simulink library "ddm"  (R2021b)
settings: Solver=VariableStepAuto  StartTime=0.0  StopTime=10.0  RelTol=1e-3
undefined symbols (not defined in the file or in its folder): ADDM_FrTMTqDev_X_Nm, ADDM_RrTMTqDev_X_Nm, ENUM_ADASACCSTA_ERROR, ENUM_ADASACCSTA_OFF, ENUM_ADASACCSTA_STANDBY, ENUM_ALLOWMOV_ALLOWREADY, ENUM_APS, ENUM_BRKSTA_ERROR, ENUM_BRKSTA_OFF, ENUM_BRKSTA_ON, ENUM_BRKSW_INVALID, ENUM_BRKSW_OFF, ENUM_BRKSW_ON, ENUM_CHGPREACTERRSTA_OBCPRE, ENUM_DCDCFAULTSTA_ANYFAULTLV1, ENUM_DCDCFAULTSTA_ANYFAULTLV2, ENUM_DRIVETRAIN_AWD, ENUM_DRIVETRAIN_FWD, ENUM_DRIVETRAIN_RWD, ENUM_EDUDRTSTA_NORMAL, ENUM_EPBSTA_APPLIED, ENUM_EPBSTA_RELEASED, ENUM_ESCAPSSta_APSUNAVAILABLE, ENUM_GEARACTUALPOSN_INVALID, ENUM_GEARACTUALPOSN_P, ENUM_HVBATTREADYPRE_READY, ENUM_MCUWARN_LV0, ENUM_MCUWARN_LV1, ENUM_MCUWARN_LV2, ENUM_MCUWARN_LV3, ENUM_MCUWARN_NOERROR, ENUM_OBCFAULTSTA_ANYFAULT, ENUM_PAS_R2F2, ENUM_PDFAULT_BATTPDFAIL, ENUM_PDFAULT_DCDCDISABLE, ENUM_PDFAULT_MCUDISABLE, ENUM_PDFAULT_MCUDISCHRG, ENUM_POWERSTA_OFF, ENUM_POWERSTA_ON, ENUM_POWERSTA_READY, ENUM_POWERSTA_STANDBY, ENUM_PRESSINDI_LOW, ENUM_PUFAULT_BATTUPFAIL, ENUM_PUFAULT_DCDCENABLEFAIL, ENUM_PUFAULT_PRECHRGCHKFAIL, ENUM_PUFAULT_SAFETYCHKFAIL, ENUM_PUSTATE_COMPLETED, ENUM_PWRSTASW_OFF, ENUM_PWRSTASW_OFFA, ENUM_PWRSTASW_OFFCHVCHRG, ENUM_PWRSTASW_OFFCLVCHRG, ENUM_PWRSTASW_ON, ENUM_PWRSTASW_ONHVCHRG, ENUM_PWRSTASW_READY, ENUM_PWRSTASW_STANDBY, ENUM_RAPSErrWarnSta_NORMAL, ENUM_RAPSErrWarnSta_RAPSERRLV1, ENUM_SHIFTCOMMAND_P, ENUM_SHIFTERERRSTA_PBUTTONFAILURE, ENUM_VEHMALFUNLV_2ND ... (+463)
libraries: hcu_lib x529, $bdroot x5, simulink x4
(part 6 of 25)

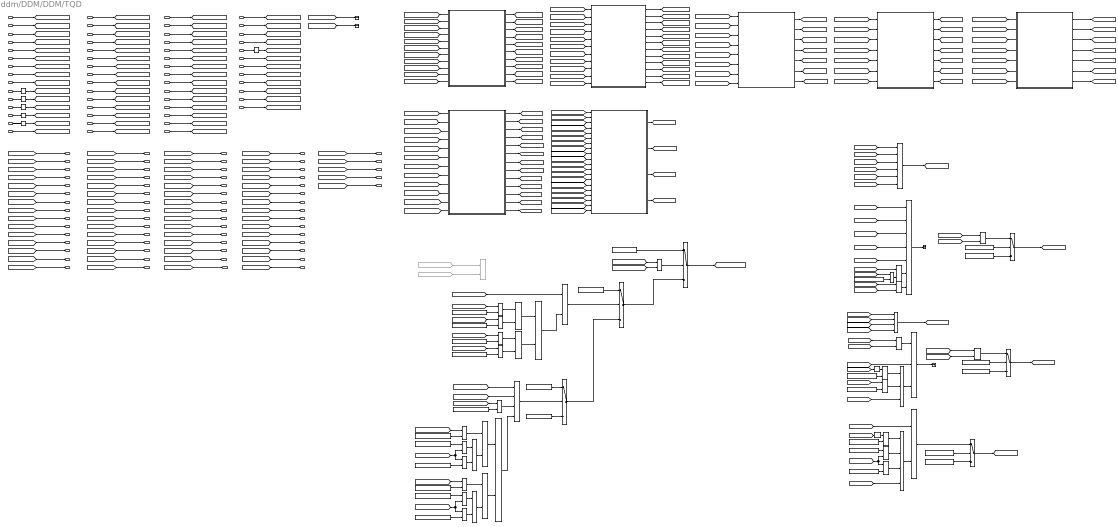
== system ddm/DDM/DDM/TQD ==
  note: VDDM_EPB1Err_flg
  note: Shifeter Error lamp Signal
  note: Three-electrical warning
  note: Warning lamp Signal
  note: RAPS Signal error
  VPMM_SysPwrSta_enum : Inport
  VINP_AccelPedal1Vol_V : Inport  Port=2
  VINP_AccelPedal2Vol_V : Inport  Port=3
  VDHP_EAPS12RangeSta_enum : Inport  Port=4
  VDHP_EAPCRBAD_flg : Inport  Port=5
  task_time_s : Inport  Port=6
  DTC_clear_request : Inport  Port=7
  No_CAN3_BUS_OFF : Inport  Port=8
  No_CAN1_BUS_OFF : Inport  Port=9
  VINP_CANMsgValidMCUNF1_flg : Inport  Port=10
  VINP_CANMsgValidMCUNR1_flg : Inport  Port=11
  VINP_CANMsgValidShifter1_flg : Inport  Port=12
  VINP_CANMsgValidESC1_flg : Inport  Port=13
  VINP_CANMsgValidESC5_flg : Inport  Port=14
  VDDM_MCUNF1RCErr_flg : Inport  Port=15
  VDDM_MCUNF1CSErr_flg : Inport  Port=16
  VDDM_MCUNR1RCErr_flg : Inport  Port=17
  VDDM_MCUNR1CSErr_flg : Inport  Port=18
  VDDM_Shifter1RCErr_flg : Inport  Port=19
  VDDM_Shifter1CSErr_flg : Inport  Port=20
  VDDM_ESC1RCErr_flg : Inport  Port=21
  VDDM_ESC1CSErr_flg : Inport  Port=22
  VDDM_ESC5RCErr_flg : Inport  Port=23
  VDDM_ESC5CSErr_flg : Inport  Port=24
  VINP_FrEDUDrtStaNidec_flg : Inport  Port=25
  VINP_VehSpeed_kph : Inport  Port=26
  VINP_FrEDURealTMTqNidec_Nm : Inport  Port=27
  VTQR_FrTMTqReq_Nm : Inport  Port=28
  VINP_RrEDUDrtStaNidec_flg : Inport  Port=29
  VINP_RrEDURealTMTqNidec_Nm : Inport  Port=30
  VTQR_RrTMTqReq_Nm : Inport  Port=31
  VINP_MCUWarnFNidec_enum : Inport  Port=32
  VINP_MCUWarnRNidec_enum : Inport  Port=33
  VINP_Pedal1Ref5V_V : Inport  Port=34
  VINP_Pedal2Ref5V_V : Inport  Port=35
  VINP_HVBattSOC_pct : Inport  Port=36
  VDDM_AuxBattVolV_V : Inport  Port=37
  VTQD_ActParkRequest_flg : Inport  Port=38
  VINP_EPBSta_enum : Inport  Port=39
  VINP_ShifterHandleCmd_enum : Inport  Port=40
  VINP_BMSWarn4_flg : Inport  Port=41
  VINP_BMSWarn5_flg : Inport  Port=42
  VINP_BMSWarn6_flg : Inport  Port=43
  VINP_BMSWarn7_flg : Inport  Port=44
  VINP_BMSWarn8_flg : Inport  Port=45
  VINP_DCDCFaultSta_enum : Inport  Port=46
  VPMM_DrivetrainSelect_enum : Inport  Port=47
  VTQD_GearActualPosn_enum : Inport  Port=48
  VINP_EPBErrSta_enum : Inport  Port=49
  VINP_CANMsgValidEPB1_flg : Inport  Port=50
  VDDM_EPB1RCErr_flg : Inport  Port=51
  VDDM_EPB1CSErr_flg : Inport  Port=52
  VDHP_EAPS1BAD_flg : Inport  Port=53
  VDHP_EAPS2BAD_flg : Inport  Port=54
  VDDM_C3BMS1LCCFS_flg : Inport  Port=55
  VDDM_VCURAPSErrLv2_flg : Inport  Port=56
  VVMC_APSActive_flg : Inport  Port=57
  APS_DDM : Subsystem
  Constant : Constant  Value=KDDM_SysErrShifterErrSW_flg
  Constant1 : Constant  Value=ENUM_DRIVETRAIN_FWD
  Constant10 : Constant  Value=ENUM_MCUWARN_LV3
  Constant11 : Constant  Value=ENUM_VEHMALFUNLV_3RD
  Constant12 : Constant  Value=ENUM_VEHMALFUNLV_4TH
  Constant{13..14,18..19,88} (5 alike) : Constant  Value=ENUM_GEARACTUALPOSN_P
  Constant15 : Constant  Value=ENUM_VEHMALFUNLV_2ND
  Constant16 : Constant  Value=ENUM_VEHMALFUNLV_NORMAL
  Constant17 : Constant  Value=ENUM_DCDCFAULTSTA_ANYFAULTLV2
  Constant2 : Constant  Value=ENUM_MCUWARN_LV1
  Constant20 : Constant  Value=ENUM_GEARACTUALPOSN_INVALID
  Constant21 : Constant  Value=FALSE
  Constant22 : Constant  Value=KDDM_EPBErrPopupSW_flg
  Constant23 : Constant  Value=FALSE
  Constant24 : Constant  Value=KDDM_DisengagePFailSW_flg
  Constant25 : Constant  Value=FALSE
  Constant3 : Constant  Value=ENUM_MCUWARN_LV2
  Constant4 : Constant  Value=ENUM_DRIVETRAIN_RWD
  Constant5 : Constant  Value=ENUM_MCUWARN_LV1
  Constant6 : Constant  Value=ENUM_MCUWARN_LV2
  Constant7 : Constant  Value=ENUM_DRIVETRAIN_FWD
  Constant8 : Constant  Value=ENUM_DRIVETRAIN_RWD
  Constant9 : Constant  Value=ENUM_MCUWARN_LV3
  Delay1 : Delay  DelayLength=1
  Delay2 : Delay  DelayLength=1
  EPB : Subsystem
  ESC1_DDM : Subsystem
  ESC5_DDM : Subsystem
  Equal{,1,5,8,11,15..16} (7 alike) : RelationalOperator  Operator=~=  OutDataTypeStr=boolean  RndMeth=Simplest
  Equal{2..4,6..7,9..10,12..14} (10 alike) : RelationalOperator  Operator===  OutDataTypeStr=boolean  RndMeth=Simplest
  From112 : From  Commented=on  GotoTag=VDDM_MCUNR1NoComCFS_flg
  From176 : From  Commented=on  GotoTag=VDDM_C3BMS1LCCFS_flg
  Logical Operator{,1,3..5,8} (6 alike) : Logic  Operator=NOT  AllPortsSameDT=off  OutDataTypeStr=boolean
  Logical Operator{2,10..13} (5 alike) : Logic  AllPortsSameDT=off  OutDataTypeStr=boolean
  Logical Operator6 : Logic  Inputs=3  AllPortsSameDT=off  OutDataTypeStr=boolean
  Logical Operator7 : Logic  Operator=OR  Inputs=4  AllPortsSameDT=off  OutDataTypeStr=boolean
  Logical Operator9 : Logic  Inputs=4  AllPortsSameDT=off  OutDataTypeStr=boolean
  MCU1_Nidec_DDM : Subsystem
  MCU_Nidec_DDM : Subsystem
  OR : Logic  Operator=OR  Inputs=6  AllPortsSameDT=off  OutDataTypeStr=boolean
  OR1 : Logic  Operator=OR  Inputs=7  AllPortsSameDT=off  OutDataTypeStr=boolean
  OR{4,6..7,9..10,12,14} (7 alike) : Logic  Operator=OR  AllPortsSameDT=off  OutDataTypeStr=boolean
  OR{5,8,11,13} (4 alike) : Logic  AllPortsSameDT=off  OutDataTypeStr=boolean
  OR15 : Logic  Commented=on  Operator=OR  AllPortsSameDT=off  OutDataTypeStr=boolean
  OR2 : Logic  Operator=OR  Inputs=3  AllPortsSameDT=off  OutDataTypeStr=boolean
  OR3 : Logic  Operator=OR  Inputs=4  AllPortsSameDT=off  OutDataTypeStr=boolean
  Shifter1_DDM : Subsystem
  Switch : Switch  Criteria=u2 > Threshold
  Switch1 : Switch  Criteria=u2 ~= 0
  Switch2 : Switch  Criteria=u2 ~= 0
  Switch3 : Switch  Criteria=u2 > Threshold
  Switch4 : Switch  Criteria=u2 > Threshold
  Switch6 : Switch  Criteria=u2 ~= 0
  Terminator{,1..3} (4 alike) : Terminator
  VDDM_APS1SigOoRDTC_raw32 : Outport
  VDDM_APS2SigOoRDTC_raw32 : Outport  Port=2
  VDDM_APSCorrErrDTC_raw32 : Outport  Port=3
  VDDM_MCUF1NoComDTC_raw32 : Outport  Port=4
  VDDM_MCUR1NoComDTC_raw32 : Outport  Port=5
  VDDM_Shifter1NoComDTC_raw32 : Outport  Port=6
  VDDM_ESC1NoComDTC_raw32 : Outport  Port=7
  VDDM_ESC5NoComDTC_raw32 : Outport  Port=8
  VDDM_MCUF1RCErrDTC_raw32 : Outport  Port=9
  VDDM_MCUR1RCErrDTC_raw32 : Outport  Port=10
  VDDM_MCUF1CSErrDTC_raw32 : Outport  Port=11
  VDDM_MCUR1CSErrDTC_raw32 : Outport  Port=12
  VDDM_Shifter1RCErrDTC_raw32 : Outport  Port=13
  VDDM_Shifter1CSErrDTC_raw32 : Outport  Port=14
  VDDM_ESC1RCErrDTC_raw32 : Outport  Port=15
  VDDM_ESC1CSErrDTC_raw32 : Outport  Port=16
  VDDM_ESC5RCErrDTC_raw32 : Outport  Port=17
  VDDM_ESC5CSErrDTC_raw32 : Outport  Port=18
  VDDM_FrMCUTqErrDTC_raw32 : Outport  Port=19
  VDDM_RrMCUTqErrDTC_raw32 : Outport  Port=20
  VDDM_MCUNF1NoComCFS_flg : Outport  Port=21
  VDDM_MCUNF1RCErrCFS_flg : Outport  Port=22
  VDDM_MCUNF1CSErrCFS_flg : Outport  Port=23
  VDDM_MCUNR1NoComCFS_flg : Outport  Port=24
  VDDM_MCUNR1RCErrCFS_flg : Outport  Port=25
  VDDM_MCUNR1CSErrCFS_flg : Outport  Port=26
  VDDM_ESC1NoComCFS_flg : Outport  Port=27
  VDDM_ESC1RCErrCFS_flg : Outport  Port=28
  VDDM_ESC1CSErrCFS_flg : Outport  Port=29
  VDDM_ESC5NoComCFS_flg : Outport  Port=30
  VDDM_ESC5RCErrCFS_flg : Outport  Port=31
  VDDM_ESC5CSErrCFS_flg : Outport  Port=32
  VDDM_5vAPS1OoRDTC_raw32 : Outport  Port=33
  VDDM_5vAPS2OoRDTC_raw32 : Outport  Port=34
  VDDM_EDriveSysErrTQD_flg : Outport  Port=35
  VDDM_EDriveSysErrShifterErr_flg : Outport  Port=36
  VDDM_EngagePFail_flg : Outport  Port=37
  VDDM_VehMalfunLevelTmp_enum : Outport  Port=38
  VDDM_EPBLockTODTC_raw32 : Outport  Port=39
  VDDM_EPBUnlockTODTC_raw32 : Outport  Port=40
  VDDM_EPB1NoComDTC_raw32 : Outport  Port=41
  VDDM_EPB1RCErrDTC_raw32 : Outport  Port=42
  VDDM_EPB1CSErrDTC_raw32 : Outport  Port=43
  VDDM_EPBSigErrDTC_raw32 : Outport  Port=44
  VDDM_5vAPS1OoRCFS_flg : Outport  Port=45
  VDDM_5vAPS2OoRCFS_flg : Outport  Port=46
  VDDM_APS1SigOoRCFS_flg : Outport  Port=47
  VDDM_APS2SigOoRCFS_flg : Outport  Port=48
  VDDM_APSCorrErrCFS_flg : Outport  Port=49
  VDDM_Shifter1NoComCFS_flg : Outport  Port=50
  VDDM_Shifter1RCErrCFS_flg : Outport  Port=51
  VDDM_Shifter1CSErrCFS_flg : Outport  Port=52
  VDDM_EPBSigErrCFS_flg : Outport  Port=53
  VDDM_EPB1NoComCFS_flg : Outport  Port=54
  VDDM_EPB1RCErrCFS_flg : Outport  Port=55
  VDDM_EPB1CSErrCFS_flg : Outport  Port=56
  VDDM_EPBLockTOCFS_flg : Outport  Port=57
  VDDM_EPBUnlockTOCFS_flg : Outport  Port=58
  VDDM_FrMCUNTqErrCFS_flg : Outport  Port=59
  VDDM_RrMCUNTqErrCFS_flg : Outport  Port=60
  VDDM_DisengagePFail_flg : Outport  Port=61
  VDDM_Shifter1Err_flg : Outport  Port=62
  VDDM_EPB1Err_flg : Outport  Port=63
  VDDM_ESC5Err_flg : Outport  Port=64
  VDDM_ESC1Err_flg : Outport  Port=65
  wires:
  VINP_ShifterHandleCmd_enum/1 -> [VINP_ShifterHandleCmd_enum]
  VINP_EPBSta_enum/1 -> [VINP_EPBSta_enum]
  VTQD_ActParkRequest_flg/1 -> [VTQD_ActParkRequest_flg]
  VDDM_AuxBattVolV_V/1 -> [VDDM_AuxBattVolV_V]
  VINP_HVBattSOC_pct/1 -> [VINP_HVBattSOC_pct]
  [VINP_Pedal2Ref5V_V] -> APS_DDM/7(VINP_Pedal2Ref5V_V)
  [VINP_Pedal1Ref5V_V] -> APS_DDM/6(VINP_Pedal1Ref5V_V)
  VINP_Pedal2Ref5V_V/1 -> [VINP_Pedal2Ref5V_V]
  VINP_Pedal1Ref5V_V/1 -> [VINP_Pedal1Ref5V_V]
  [VDDM_MCUNR1RCErrCFS_flg] -> MCU_Nidec_DDM/12(VDDM_MCUNR1RCErrCFS_flg)
  [VDDM_MCUNF1RCErrCFS_flg] -> MCU_Nidec_DDM/5(VDDM_MCUNF1RCErrCFS_flg)
  [VDDM_MCUNF1CSErrCFS_flg] -> MCU_Nidec_DDM/6(VDDM_MCUNF1CSErrCFS_flg)
  [No_CAN3_BUS_OFF] -> MCU_Nidec_DDM/3(No_CAN3_BUS_OFF)
  [VINP_MCUWarnFNidec_enum] -> MCU_Nidec_DDM/17(VINP_MCUWarnFNidec_enum)
  [VINP_RrEDUDrtStaNidec_flg] -> MCU_Nidec_DDM/14(VINP_RrEDUDrtStaNidec_flg)
  [VDDM_MCUNR1CSErrCFS_flg] -> MCU_Nidec_DDM/13(VDDM_MCUNR1CSErrCFS_flg)
  [VPMM_SysPwrSta_enum] -> MCU_Nidec_DDM/2(VPMM_SysPwrSta_enum)
  [VDDM_MCUNF1NoComCFS_flg] -> MCU_Nidec_DDM/4(VDDM_MCUNF1NoComCFS_flg)
  [VTQR_FrTMTqReq_Nm] -> MCU_Nidec_DDM/10(VTQR_FrTMTqReq_Nm)
  [task_time_s] -> MCU_Nidec_DDM/1(task_time_s)
  [VTQR_RrTMTqReq_Nm] -> MCU_Nidec_DDM/16(VTQR_RrTMTqReq_Nm)
  [VINP_FrEDUDrtStaNidec_flg] -> MCU_Nidec_DDM/8(VINP_FrEDUDrtStaNidec_flg)
  [VINP_FrEDURealTMTqNidec_Nm] -> MCU_Nidec_DDM/9(VINP_FrEDURealTMTqNidec_Nm)
  [VINP_RrEDURealTMTqNidec_Nm] -> MCU_Nidec_DDM/15(VINP_RrEDURealTMTqNidec_Nm)
  [DTC_clear_request] -> MCU_Nidec_DDM/19(DTC_clear_request)
  [VDDM_MCUNR1NoComCFS_flg] -> MCU_Nidec_DDM/11(VDDM_MCUNR1NoComCFS_flg)
  [VINP_MCUWarnRNidec_enum] -> MCU_Nidec_DDM/18(VINP_MCUWarnRNidec_enum)
  [VINP_VehSpeed_kph] -> MCU_Nidec_DDM/7(VINP_VehSpeed_kph)
  [VDDM_MCUNF1RCErrCFS_flg] -> VDDM_MCUNF1RCErrCFS_flg/1
  [VDDM_MCUNR1RCErrCFS_flg] -> VDDM_MCUNR1RCErrCFS_flg/1
  [VDDM_MCUNR1NoComCFS_flg] -> VDDM_MCUNR1NoComCFS_flg/1
  [VDDM_MCUNF1CSErrCFS_flg] -> VDDM_MCUNF1CSErrCFS_flg/1
  [VDDM_MCUNR1CSErrCFS_flg] -> VDDM_MCUNR1CSErrCFS_flg/1
  [VDDM_MCUNF1NoComCFS_flg] -> VDDM_MCUNF1NoComCFS_flg/1
  MCU1_Nidec_DDM/11(VDDM_MCUNR1RCErrCFS_flg) -> [VDDM_MCUNR1RCErrCFS_flg]
  MCU1_Nidec_DDM/7(VDDM_MCUNF1NoComCFS_flg) -> [VDDM_MCUNF1NoComCFS_flg]
  MCU1_Nidec_DDM/10(VDDM_MCUNR1NoComCFS_flg) -> [VDDM_MCUNR1NoComCFS_flg]
  MCU1_Nidec_DDM/9(VDDM_MCUNF1CSErrCFS_flg) -> [VDDM_MCUNF1CSErrCFS_flg]
  MCU1_Nidec_DDM/8(VDDM_MCUNF1RCErrCFS_flg) -> [VDDM_MCUNF1RCErrCFS_flg]
  MCU1_Nidec_DDM/12(VDDM_MCUNR1CSErrCFS_flg) -> [VDDM_MCUNR1CSErrCFS_flg]
  VINP_MCUWarnRNidec_enum/1 -> [VINP_MCUWarnRNidec_enum]
  VINP_MCUWarnFNidec_enum/1 -> [VINP_MCUWarnFNidec_enum]
  VINP_VehSpeed_kph/1 -> [VINP_VehSpeed_kph]
  VINP_RrEDUDrtStaNidec_flg/1 -> [VINP_RrEDUDrtStaNidec_flg]
  VTQR_FrTMTqReq_Nm/1 -> [VTQR_FrTMTqReq_Nm]
  VINP_FrEDURealTMTqNidec_Nm/1 -> [VINP_FrEDURealTMTqNidec_Nm]
  VTQR_RrTMTqReq_Nm/1 -> [VTQR_RrTMTqReq_Nm]
  VINP_FrEDUDrtStaNidec_flg/1 -> [VINP_FrEDUDrtStaNidec_flg]
  VINP_RrEDURealTMTqNidec_Nm/1 -> [VINP_RrEDURealTMTqNidec_Nm]
  VDDM_ESC5RCErr_flg/1 -> [VDDM_ESC5RCErr_flg]
  VDDM_ESC5CSErr_flg/1 -> [VDDM_ESC5CSErr_flg]
  [VDDM_ESC5CSErr_flg] -> ESC5_DDM/6(VDDM_ESC5CSErr_flg)
  [VDDM_ESC5RCErr_flg] -> ESC5_DDM/5(VDDM_ESC5RCErr_flg)
  VDDM_ESC1RCErr_flg/1 -> [VDDM_ESC1RCErr_flg]
  VDDM_ESC1CSErr_flg/1 -> [VDDM_ESC1CSErr_flg]
  VDDM_Shifter1CSErr_flg/1 -> [VDDM_Shifter1CSErr_flg]
  VDDM_Shifter1RCErr_flg/1 -> [VDDM_Shifter1RCErr_flg]
  VDDM_MCUNF1RCErr_flg/1 -> [VDDM_MCUNF1RCErr_flg]
  VDDM_MCUNF1CSErr_flg/1 -> [VDDM_MCUNF1CSErr_flg]
  VDDM_MCUNR1CSErr_flg/1 -> [VDDM_MCUNR1CSErr_flg]
  VDDM_MCUNR1RCErr_flg/1 -> [VDDM_MCUNR1RCErr_flg]
  [VDDM_Shifter1CSErr_flg] -> Shifter1_DDM/6(VDDM_Shifter1CSErr_flg)
  [VDDM_Shifter1RCErr_flg] -> Shifter1_DDM/5(VDDM_Shifter1RCErr_flg)
  [VDDM_MCUNR1CSErr_flg] -> MCU1_Nidec_DDM/9(VDDM_MCUNR1CSErr_flg)
  [VDDM_MCUNR1RCErr_flg] -> MCU1_Nidec_DDM/8(VDDM_MCUNR1RCErr_flg)
  [VDDM_MCUNF1CSErr_flg] -> MCU1_Nidec_DDM/7(VDDM_MCUNF1CSErr_flg)
  [VDDM_MCUNF1RCErr_flg] -> MCU1_Nidec_DDM/6(VDDM_MCUNF1RCErr_flg)
  Logical Operator5/1 -> [VDDM_MCUNF1NoCom_flg]
  Logical Operator4/1 -> [VDDM_MCUNR1NoCom_flg]
  Logical Operator3/1 -> [VDDM_Shifter1NoCom_flg]
  Logical Operator1/1 -> [VDDM_ESC1NoCom_flg]
  Logical Operator/1 -> [VDDM_ESC5NoCom_flg]
  VINP_CANMsgValidESC5_flg/1 -> Logical Operator/1
  VINP_CANMsgValidESC1_flg/1 -> Logical Operator1/1
  VINP_CANMsgValidShifter1_flg/1 -> Logical Operator3/1
  VINP_CANMsgValidMCUNR1_flg/1 -> Logical Operator4/1
  VINP_CANMsgValidMCUNF1_flg/1 -> Logical Operator5/1
  No_CAN1_BUS_OFF/1 -> [No_CAN1_BUS_OFF]
  No_CAN3_BUS_OFF/1 -> [No_CAN3_BUS_OFF]
  [DTC_clear_request] -> ESC5_DDM/7(DTC_clear_request)
  [VDDM_ESC5NoCom_flg] -> ESC5_DDM/4(VDDM_ESC5NoCom_flg)
  [No_CAN1_BUS_OFF] -> ESC5_DDM/3(No_CAN1_BUS_OFF)
  [VPMM_SysPwrSta_enum] -> ESC5_DDM/2(VPMM_SysPwrSta_enum)
  [task_time_s] -> ESC5_DDM/1(task_time_s)
  [No_CAN1_BUS_OFF] -> ESC1_DDM/3(No_CAN1_BUS_OFF)
  [VPMM_SysPwrSta_enum] -> ESC1_DDM/2(VPMM_SysPwrSta_enum)
  [task_time_s] -> ESC1_DDM/1(task_time_s)
  [DTC_clear_request] -> Shifter1_DDM/7(DTC_clear_request)
  [VDDM_Shifter1NoCom_flg] -> Shifter1_DDM/4(VDDM_Shifter1NoCom_flg)
  [No_CAN3_BUS_OFF] -> Shifter1_DDM/3(No_CAN3_BUS_OFF)
  [VPMM_SysPwrSta_enum] -> Shifter1_DDM/2(VPMM_SysPwrSta_enum)
  [DTC_clear_request] -> MCU1_Nidec_DDM/10(DTC_clear_request)
  [VDDM_MCUNR1NoCom_flg] -> MCU1_Nidec_DDM/5(VDDM_MCUNR1NoCom_flg)
  [VDDM_MCUNF1NoCom_flg] -> MCU1_Nidec_DDM/4(VDDM_MCUNF1NoCom_flg)
  [No_CAN3_BUS_OFF] -> MCU1_Nidec_DDM/3(No_CAN3_BUS_OFF)
  [VPMM_SysPwrSta_enum] -> MCU1_Nidec_DDM/2(VPMM_SysPwrSta_enum)
  [task_time_s] -> Shifter1_DDM/1(task_time_s)
  [task_time_s] -> MCU1_Nidec_DDM/1(task_time_s)
  DTC_clear_request/1 -> [DTC_clear_request]
  task_time_s/1 -> [task_time_s]
  [VDHP_EAPS12RangeSta_enum] -> APS_DDM/4(VDHP_EAPS12RangeSta_enum)
  [VINP_AccelPedal2Vol_V] -> APS_DDM/3(VINP_AccelPedal2Vol_V)
  [VINP_AccelPedal1Vol_V] -> APS_DDM/2(VINP_AccelPedal1Vol_V)
  [VPMM_SysPwrSta_enum] -> APS_DDM/1(VPMM_SysPwrSta_enum)
  [VDHP_EAPCRBAD_flg] -> APS_DDM/5(VDHP_EAPCRBAD_flg)
  VPMM_SysPwrSta_enum/1 -> [VPMM_SysPwrSta_enum]
  VINP_AccelPedal1Vol_V/1 -> [VINP_AccelPedal1Vol_V]
  VDHP_EAPCRBAD_flg/1 -> [VDHP_EAPCRBAD_flg]
  VDHP_EAPS12RangeSta_enum/1 -> [VDHP_EAPS12RangeSta_enum]
  VINP_AccelPedal2Vol_V/1 -> [VINP_AccelPedal2Vol_V]
  Shifter1_DDM/4(VDDM_Shifter1NoComCFS_flg) -> [VDDM_Shifter1NoComCFS_flg]
  Shifter1_DDM/5(VDDM_Shifter1RCErrCFS_flg) -> [VDDM_Shifter1RCErrCFS_flg]
  Shifter1_DDM/6(VDDM_Shifter1CSErrCFS_flg) -> [VDDM_Shifter1CSErrCFS_flg]
  Switch/1 -> [VDDM_EDriveSysErrShifterErr_flg]  "VDDM_EDriveSysErrShifterErr_flg"
  [VDDM_Shifter1RCErrCFS_flg] -> OR1/2
  [VDDM_Shifter1NoComCFS_flg] -> OR1/1
  [VDDM_Shifter1CSErrCFS_flg] -> OR1/3
  [VDDM_EPBLockTOCFS_flg] -> OR1/4
  [VDDM_EPBUnlockTOCFS_flg] -> OR1/5
  [VDDM_Shifter1RCErrCFS_flg] -> OR/2
  [VDDM_Shifter1CSErrCFS_flg] -> OR/3
  [VDDM_Shifter1NoComCFS_flg] -> OR/1
  [VDDM_EPBLockTOCFS_flg] -> OR/4
  [VDDM_EPBUnlockTOCFS_flg] -> OR/5
  Switch3/1 -> [VDDM_EngagePFail_flg]  "VDDM_EngagePFail_flg"
  VINP_BMSWarn4_flg/1 -> [VINP_BMSWarn4_flg]
  VINP_BMSWarn5_flg/1 -> [VINP_BMSWarn5_flg]
  VINP_BMSWarn6_flg/1 -> [VINP_BMSWarn6_flg]
  VINP_BMSWarn7_flg/1 -> [VINP_BMSWarn7_flg]
  VINP_BMSWarn8_flg/1 -> [VINP_BMSWarn8_flg]
  VINP_DCDCFaultSta_enum/1 -> [VINP_DCDCFaultSta_enum]
  VPMM_DrivetrainSelect_enum/1 -> [VPMM_DrivetrainSelect_enum]
  [VDDM_VehMalfunLevelTmp_enum] -> VDDM_VehMalfunLevelTmp_enum/1
  [VPMM_DrivetrainSelect_enum] -> MCU1_Nidec_DDM/11(VPMM_DrivetrainSelect_enum)
  [VTQD_GearActualPosn_enum] -> Shifter1_DDM/8(VINP_ShifterHandleCmd_enum)
  VTQD_GearActualPosn_enum/1 -> [VTQD_GearActualPosn_enum]
  [VDDM_ESC1NoCom_flg] -> ESC1_DDM/4(VDDM_ESC1NoCom_flg)
  [VDDM_ESC1RCErr_flg] -> ESC1_DDM/5(VDDM_ESC1RCErr_flg)
  [VDDM_ESC1CSErr_flg] -> ESC1_DDM/6(VDDM_ESC1CSErr_flg)
  [DTC_clear_request] -> ESC1_DDM/7(DTC_clear_request)
  [VTQD_ActParkRequest_flg] -> EPB/5(VTQD_ActParkRequest_flg)
  EPB/10(VDDM_EPB1NoComCFS_flg) -> [VDDM_EPB1NoComCFS_flg]
  [DTC_clear_request] -> EPB/9(DTC_clear_request)
  [No_CAN1_BUS_OFF] -> EPB/1(NO_CAN1_BUS_OFF)
  [VDDM_EPB1NoCom_flg] -> EPB/10(VDDM_EPB1NoCom_flg)
  [task_time_s] -> EPB/8(task_time_s)
  [VPMM_SysPwrSta_enum] -> EPB/4(VPMM_SysPwrSta_enum)
  EPB/3(VDDM_EPBLockTOCFS_flg) -> [VDDM_EPBLockTOCFS_flg]
  EPB/4(VDDM_EPBUnlockTOCFS_flg) -> [VDDM_EPBUnlockTOCFS_flg]
  EPB/9(VDDM_EPBSigErrCFS_flg) -> [VDDM_EPBSigErrCFS_flg]
  EPB/11(VDDM_EPB1RCErrCFS_flg) -> [VDDM_EPB1RCErrCFS_flg]
  [VINP_EPBSta_enum] -> EPB/6(VINP_EPBSta_enum)
  [VTQD_GearActualPosn_enum] -> EPB/2(VTQD_GearActualPosn_enum)
  [VDDM_EPB1RCErr_flg] -> EPB/11(VDDM_EPB1RCErr_flg)
  [VINP_EPBErrSta_enum] -> EPB/3(VINP_EPBErrSta_enum)
  [VDDM_EPB1CSErr_flg] -> EPB/12(VDDM_EPB1CSErr_flg)
  EPB/12(VDDM_EPB1CSErrCFS_flg) -> [VDDM_EPB1CSErrCFS_flg]
  [VINP_ShifterHandleCmd_enum] -> EPB/7(VINP_ShifterHandleCmd_enum)
  VINP_EPBErrSta_enum/1 -> [VINP_EPBErrSta_enum]
  VINP_CANMsgValidEPB1_flg/1 -> Logical Operator8/1
  VDDM_EPB1RCErr_flg/1 -> [VDDM_EPB1RCErr_flg]
  VDDM_EPB1CSErr_flg/1 -> [VDDM_EPB1CSErr_flg]
  Logical Operator8/1 -> [VDDM_EPB1NoCom_flg]
  [VPMM_DrivetrainSelect_enum] -> MCU_Nidec_DDM/20(VPMM_DrivetrainSelect_enum)
  MCU_Nidec_DDM/3(VDDM_FrMCUNTqErrCFS_flg) -> [VDDM_FrMCUNTqErrCFS_flg]
  MCU_Nidec_DDM/4(VDDM_RrMCUNTqErrCFS_flg) -> [VDDM_RrMCUNTqErrCFS_flg]
  [task_time_s] -> APS_DDM/8(task_time_s)
  [DTC_clear_request] -> APS_DDM/9(DTC_clear_request)
  [VDHP_EAPS1BAD_flg] -> APS_DDM/10(VDHP_EAPS1BAD_flg)
  [VDHP_EAPS2BAD_flg] -> APS_DDM/11(VDHP_EAPS2BAD_flg)
  VDHP_EAPS2BAD_flg/1 -> [VDHP_EAPS2BAD_flg]
  VDHP_EAPS1BAD_flg/1 -> [VDHP_EAPS1BAD_flg]
  APS_DDM/6(VDDM_5vAPS1OoRCFS_flg) -> [VDDM_5vAPS1OoRCFS_flg]
  APS_DDM/7(VDDM_5vAPS2OoRCFS_flg) -> [VDDM_5vAPS2OoRCFS_flg]
  APS_DDM/10(VDDM_APSCorrErrCFS_flg) -> [VDDM_APSCorrErrCFS_flg]
  APS_DDM/8(VDDM_APS1SigOoRCFS_flg) -> [VDDM_APS1SigOoRCFS_flg]
  APS_DDM/9(VDDM_APS2SigOoRCFS_flg) -> [VDDM_APS2SigOoRCFS_flg]
  [VDDM_5vAPS2OoRCFS_flg] -> VDDM_5vAPS2OoRCFS_flg/1
  [VDDM_APS1SigOoRCFS_flg] -> VDDM_APS1SigOoRCFS_flg/1
  [VDDM_5vAPS1OoRCFS_flg] -> VDDM_5vAPS1OoRCFS_flg/1
  [VDDM_APS2SigOoRCFS_flg] -> VDDM_APS2SigOoRCFS_flg/1
  [VDDM_APSCorrErrCFS_flg] -> VDDM_APSCorrErrCFS_flg/1
  [VDDM_Shifter1NoComCFS_flg] -> VDDM_Shifter1NoComCFS_flg/1
  [VDDM_Shifter1RCErrCFS_flg] -> VDDM_Shifter1RCErrCFS_flg/1
  [VDDM_Shifter1CSErrCFS_flg] -> VDDM_Shifter1CSErrCFS_flg/1
  ESC1_DDM/4(VDDM_ESC1NoComCFS_flg) -> [VDDM_ESC1NoComCFS_flg]
  ESC1_DDM/6(VDDM_ESC1CSErrCFS_flg) -> [VDDM_ESC1CSErrCFS_flg]
  ESC1_DDM/5(VDDM_ESC1RCErrCFS_flg) -> [VDDM_ESC1RCErrCFS_flg]
  [VDDM_ESC1NoComCFS_flg] -> VDDM_ESC1NoComCFS_flg/1
  [VDDM_ESC1RCErrCFS_flg] -> VDDM_ESC1RCErrCFS_flg/1
  [VDDM_ESC1CSErrCFS_flg] -> VDDM_ESC1CSErrCFS_flg/1
  ESC5_DDM/4(VDDM_ESC5NoComCFS_flg) -> [VDDM_ESC5NoComCFS_flg]
  ESC5_DDM/5(VDDM_ESC5RCErrCFS_flg) -> [VDDM_ESC5RCErrCFS_flg]
  ESC5_DDM/6(VDDM_ESC5CSErrCFS_flg) -> [VDDM_ESC5CSErrCFS_flg]
  [VDDM_ESC5NoComCFS_flg] -> VDDM_ESC5NoComCFS_flg/1
  [VDDM_ESC5RCErrCFS_flg] -> VDDM_ESC5RCErrCFS_flg/1
  [VDDM_ESC5CSErrCFS_flg] -> VDDM_ESC5CSErrCFS_flg/1
  [VDDM_EPBSigErrCFS_flg] -> VDDM_EPBSigErrCFS_flg/1
  [VDDM_EPB1NoComCFS_flg] -> VDDM_EPB1NoComCFS_flg/1
  [VDDM_EPB1RCErrCFS_flg] -> VDDM_EPB1RCErrCFS_flg/1
  [VDDM_EPB1CSErrCFS_flg] -> VDDM_EPB1CSErrCFS_flg/1
  [VDDM_EPBLockTOCFS_flg] -> VDDM_EPBLockTOCFS_flg/1
  [VDDM_EPBUnlockTOCFS_flg] -> VDDM_EPBUnlockTOCFS_flg/1
  [VDDM_FrMCUNTqErrCFS_flg] -> VDDM_FrMCUNTqErrCFS_flg/1
  [VDDM_RrMCUNTqErrCFS_flg] -> VDDM_RrMCUNTqErrCFS_flg/1
  Constant11/1 -> Switch2/1
  OR9/1 -> OR8/2
  OR7/1 -> OR3/4
  [VINP_MCUWarnFNidec_enum] -> Equal7/1, Equal6/2
  Equal10/1 -> OR11/2
  [VINP_BMSWarn4_flg] -> OR3/1
  [VINP_BMSWarn8_flg] -> OR4/2
  Constant1/1 -> Equal1/2
  OR3/1 -> Switch6/2
  Constant17/1 -> Equal2/2
  Constant2/1 -> Equal3/1
  Constant4/1 -> Equal5/2
  Constant15/1 -> Switch6/1
  Constant7/1 -> Equal8/2
  Equal2/1 -> OR3/3
  OR6/1 -> OR5/2
  Equal1/1 -> OR5/1
  OR4/1 -> Switch1/2
  [VPMM_DrivetrainSelect_enum] -> Equal5/1
  Equal6/1 -> OR9/1
  Constant16/1 -> Switch6/3
  Equal11/1 -> OR13/1
  Constant3/1 -> Equal4/2
  Equal8/1 -> OR11/1
  Constant5/1 -> Equal6/1
  OR8/1 -> OR7/2
  Equal9/1 -> OR13/2
  Equal5/1 -> OR8/1
  [VINP_MCUWarnRNidec_enum] -> Equal4/1, Equal3/2
  OR10/1 -> Switch2/2
  Equal4/1 -> OR6/2
  OR5/1 -> OR7/1
  [VINP_BMSWarn7_flg] -> OR4/1
  Constant9/1 -> Equal10/2
  [VINP_BMSWarn5_flg] -> OR3/2
  [VPMM_DrivetrainSelect_enum] -> Equal11/1
  OR11/1 -> OR12/1
  Constant10/1 -> Equal9/2
  [VPMM_DrivetrainSelect_enum] -> Equal8/1
  Switch6/1 -> Switch2/3
  Constant8/1 -> Equal11/2
  [VINP_MCUWarnFNidec_enum] -> Equal9/1
  Switch1/1 -> [VDDM_VehMalfunLevelTmp_enum]  "VDDM_VehMalfunLevelTmp_enum"
  Switch2/1 -> Switch1/3
  Equal3/1 -> OR6/1
  OR13/1 -> OR12/2
  Constant6/1 -> Equal7/2
  [VINP_DCDCFaultSta_enum] -> Equal2/1
  Constant12/1 -> Switch1/1
  Equal7/1 -> OR9/2
  [VPMM_DrivetrainSelect_enum] -> Equal1/1
  [VINP_MCUWarnRNidec_enum] -> Equal10/1
  [VTQD_GearActualPosn_enum] -> Delay1/1
  Constant88/1 -> Equal/2
  Logical Operator6/1 -> OR2/3
  [VDDM_VCUEPBErr_flg] -> Logical Operator6/3
  [VDDM_EPBSigErrCFS_flg] -> Logical Operator7/1
  [VDDM_EPB1NoComCFS_flg] -> Logical Operator7/2
  [VDDM_EPB1RCErrCFS_flg] -> Logical Operator7/3
  [VDDM_EPB1CSErrCFS_flg] -> Logical Operator7/4
  OR/1 -> [VDDM_EDriveSysErrTQD_flg]  "VDDM_EDriveSysErrTQD_flg"
  Logical Operator7/1 -> [VDDM_VCUEPBErr_flg]  "VDDM_VCUEPBErr_flg"
  [VDDM_VCUEPBErr_flg] -> OR/6
  APS_DDM/3(VDDM_APSCorrErrDTC_raw32) -> [VDDM_APSCorrErrDTC_raw32]
  APS_DDM/2(VDDM_APS2SigOoRDTC_raw32) -> [VDDM_APS2SigOoRDTC_raw32]
  APS_DDM/1(VDDM_APS1SigOoRDTC_raw32) -> [VDDM_APS1SigOoRDTC_raw32]
  [VDDM_APS1SigOoRDTC_raw32] -> VDDM_APS1SigOoRDTC_raw32/1
  [VDDM_APS2SigOoRDTC_raw32] -> VDDM_APS2SigOoRDTC_raw32/1
  [VDDM_APSCorrErrDTC_raw32] -> VDDM_APSCorrErrDTC_raw32/1
  MCU1_Nidec_DDM/1(VDDM_MCUF1NoComDTC_raw32) -> [VDDM_MCUF1NoComDTC_raw32]
  MCU1_Nidec_DDM/2(VDDM_MCUR1NoComDTC_raw32) -> [VDDM_MCUR1NoComDTC_raw32]
  [VDDM_MCUF1NoComDTC_raw32] -> VDDM_MCUF1NoComDTC_raw32/1
  [VDDM_MCUR1NoComDTC_raw32] -> VDDM_MCUR1NoComDTC_raw32/1
  Shifter1_DDM/1(VDDM_Shifter1NoComDTC_raw32) -> [VDDM_Shifter1NoComDTC_raw32]
  ESC1_DDM/1(VDDM_ESC1NoComDTC_raw32) -> [VDDM_ESC1NoComDTC_raw32]
  ESC5_DDM/1(VDDM_ESC5NoComDTC_raw32) -> [VDDM_ESC5NoComDTC_raw32]
  [VDDM_Shifter1NoComDTC_raw32] -> VDDM_Shifter1NoComDTC_raw32/1
  [VDDM_ESC1NoComDTC_raw32] -> VDDM_ESC1NoComDTC_raw32/1
  [VDDM_ESC5NoComDTC_raw32] -> VDDM_ESC5NoComDTC_raw32/1
  MCU1_Nidec_DDM/3(VDDM_MCUF1RCErrDTC_raw32) -> [VDDM_MCUF1RCErrDTC_raw32]
  MCU1_Nidec_DDM/4(VDDM_MCUR1RCErrDTC_raw32) -> [VDDM_MCUR1RCErrDTC_raw32]
  MCU1_Nidec_DDM/5(VDDM_MCUF1CSErrDTC_raw32) -> [VDDM_MCUF1CSErrDTC_raw32]
  MCU1_Nidec_DDM/6(VDDM_MCUR1CSErrDTC_raw32) -> [VDDM_MCUR1CSErrDTC_raw32]
  [VDDM_MCUF1RCErrDTC_raw32] -> VDDM_MCUF1RCErrDTC_raw32/1
  [VDDM_MCUR1RCErrDTC_raw32] -> VDDM_MCUR1RCErrDTC_raw32/1
  [VDDM_MCUF1CSErrDTC_raw32] -> VDDM_MCUF1CSErrDTC_raw32/1
  [VDDM_MCUR1CSErrDTC_raw32] -> VDDM_MCUR1CSErrDTC_raw32/1
  Shifter1_DDM/2(VDDM_Shifter1RCErrDTC_raw32) -> [VDDM_Shifter1RCErrDTC_raw32]
  Shifter1_DDM/3(VDDM_Shifter1CSErrDTC_raw32) -> [VDDM_Shifter1CSErrDTC_raw32]
  ESC1_DDM/2(VDDM_ESC1RCErrDTC_raw32) -> [VDDM_ESC1RCErrDTC_raw32]
  [VDDM_Shifter1RCErrDTC_raw32] -> VDDM_Shifter1RCErrDTC_raw32/1
  [VDDM_Shifter1CSErrDTC_raw32] -> VDDM_Shifter1CSErrDTC_raw32/1
  [VDDM_ESC1RCErrDTC_raw32] -> VDDM_ESC1RCErrDTC_raw32/1
  ESC1_DDM/3(VDDM_ESC1CSErrDTC_raw32) -> [VDDM_ESC1CSErrDTC_raw32]
  ESC5_DDM/2(VDDM_ESC5RCErrDTC_raw32) -> [VDDM_ESC5RCErrDTC_raw32]
  ESC5_DDM/3(VDDM_ESC5CSErrDTC_raw32) -> [VDDM_ESC5CSErrDTC_raw32]
  [VDDM_ESC1CSErrDTC_raw32] -> VDDM_ESC1CSErrDTC_raw32/1
  [VDDM_ESC5RCErrDTC_raw32] -> VDDM_ESC5RCErrDTC_raw32/1
  [VDDM_ESC5CSErrDTC_raw32] -> VDDM_ESC5CSErrDTC_raw32/1
  MCU_Nidec_DDM/2(VDDM_RrMCUTqErrDTC_raw32) -> [VDDM_RrMCUTqErrDTC_raw32]
  MCU_Nidec_DDM/1(VDDM_FrMCUTqErrDTC_raw32) -> [VDDM_FrMCUTqErrDTC_raw32]
  [VDDM_FrMCUTqErrDTC_raw32] -> VDDM_FrMCUTqErrDTC_raw32/1
  [VDDM_RrMCUTqErrDTC_raw32] -> VDDM_RrMCUTqErrDTC_raw32/1
  APS_DDM/4(VDDM_5vAPS1OoRDTC_raw32) -> [VDDM_5vAPS1OoRDTC_raw32]
  APS_DDM/5(VDDM_5vAPS2OoRDTC_raw32) -> [VDDM_5vAPS2OoRDTC_raw32]
  [VDDM_5vAPS1OoRDTC_raw32] -> VDDM_5vAPS1OoRDTC_raw32/1
  [VDDM_5vAPS2OoRDTC_raw32] -> VDDM_5vAPS2OoRDTC_raw32/1
  [VDDM_EDriveSysErrTQD_flg] -> VDDM_EDriveSysErrTQD_flg/1
  [VDDM_EDriveSysErrShifterErr_flg] -> VDDM_EDriveSysErrShifterErr_flg/1
  [VDDM_EngagePFail_flg] -> VDDM_EngagePFail_flg/1
  EPB/2(VDDM_EPBUnlockTODTC_raw32) -> [VDDM_EPBUnlockTODTC_raw32]
  EPB/1(VDDM_EPBLockTODTC_raw32) -> [VDDM_EPBLockTODTC_raw32]
  EPB/5(VDDM_EPB1NoComDTC_raw32) -> [VDDM_EPB1NoComDTC_raw32]
  EPB/6(VDDM_EPB1RCErrDTC_raw32) -> [VDDM_EPB1RCErrDTC_raw32]
  EPB/8(VDDM_EPBSigErrDTC_raw32) -> [VDDM_EPBSigErrDTC_raw32]
  EPB/7(VDDM_EPB1CSErrDTC_raw32) -> [VDDM_EPB1CSErrDTC_raw32]
  [VDDM_EPBLockTODTC_raw32] -> VDDM_EPBLockTODTC_raw32/1
  [VDDM_EPBUnlockTODTC_raw32] -> VDDM_EPBUnlockTODTC_raw32/1
  [VDDM_EPB1NoComDTC_raw32] -> VDDM_EPB1NoComDTC_raw32/1
  [VDDM_EPB1RCErrDTC_raw32] -> VDDM_EPB1RCErrDTC_raw32/1
  [VDDM_EPB1CSErrDTC_raw32] -> VDDM_EPB1CSErrDTC_raw32/1
  [VDDM_EPBSigErrDTC_raw32] -> VDDM_EPBSigErrDTC_raw32/1
  [VDDM_DisengagePFail_flg] -> VDDM_DisengagePFail_flg/1
  [VINP_HVBattSOC_pct] -> Terminator/1
  [VDDM_AuxBattVolV_V] -> Terminator1/1
  Constant13/1 -> Equal12/2
  Equal12/1 -> Logical Operator2/2
  [VTQD_GearActualPosn_enum] -> Equal12/1
  Logical Operator2/1 -> OR1/6
  [VDDM_VCUEPBErr_flg] -> Logical Operator2/1
  Equal/1 -> Logical Operator6/1
  Delay1/1 -> Equal/1
  Equal13/1 -> Logical Operator6/2
  Constant14/1 -> Equal13/2
  [VTQD_GearActualPosn_enum] -> Equal13/1
  Equal15/1 -> Logical Operator9/2
  Constant19/1 -> Equal14/2
  [VDDM_VCUEPBErr_flg] -> Logical Operator9/4
  Equal14/1 -> Logical Operator9/1
  Logical Operator9/1 -> OR14/2
  Switch4/1 -> [VDDM_DisengagePFail_flg]  "VDDM_DisengagePFail_flg"
  [VTQD_GearActualPosn_enum] -> Delay2/1
  Delay2/1 -> Equal14/1
  Equal16/1 -> Logical Operator9/3
  [VTQD_GearActualPosn_enum] -> Equal15/2, Equal16/1
  Constant20/1 -> Equal16/2
  Constant18/1 -> Equal15/1
  [VDDM_EPBUnlockTOCFS_flg] -> OR14/1
  OR12/1 -> OR10/2
  [VINP_BMSWarn6_flg] -> OR10/1
  From112/1 -> OR15/1
  VDDM_C3BMS1LCCFS_flg/1 -> [VDDM_C3BMS1LCCFS_flg]
  From176/1 -> OR15/2
  Shifter1_DDM/7(VDDM_Shifter1Err_flg) -> [VDDM_Shifter1Err_flg]
  [VDDM_Shifter1Err_flg] -> VDDM_Shifter1Err_flg/1
  EPB/13(VDDM_EPB1Err_flg) -> [VDDM_EPB1Err_flg]
  [VDDM_EPB1Err_flg] -> VDDM_EPB1Err_flg/1
  ESC1_DDM/7(VDDM_ESC1Err_flg) -> [VDDM_ESC1Err_flg]
  ESC5_DDM/7(VDDM_ESC5Err_flg) -> [VDDM_ESC5Err_flg]
  [VDDM_ESC5Err_flg] -> VDDM_ESC5Err_flg/1
  [VDDM_ESC1Err_flg] -> VDDM_ESC1Err_flg/1
  [VDDM_EPBLockTOCFS_flg] -> OR2/2
  [VDDM_VCURAPSErrLv2_flg] -> Logical Operator12/1
  [VVMC_APSActive_flg] -> Logical Operator12/2
  Logical Operator12/1 -> OR2/1
  [VVMC_APSActive_flg] -> Logical Operator11/2
  [VDDM_VCURAPSErrLv2_flg] -> Logical Operator11/1
  Logical Operator11/1 -> OR1/7
  VVMC_APSActive_flg/1 -> [VVMC_APSActive_flg]
  VDDM_VCURAPSErrLv2_flg/1 -> [VDDM_VCURAPSErrLv2_flg]
  Constant/1 -> Switch/2
  Constant21/1 -> Switch/3
  Constant22/1 -> Switch3/2
  Constant23/1 -> Switch3/3
  Constant25/1 -> Switch4/3
  Constant24/1 -> Switch4/2
  OR14/1 -> Switch4/1
  [VDDM_VCURAPSErrLv2_flg] -> Logical Operator10/1
  [VVMC_APSActive_flg] -> Logical Operator10/2
  OR1/1 -> Terminator2/1
  Logical Operator10/1 -> Switch/1
  OR2/1 -> Terminator3/1
  [VVMC_APSActive_flg] -> Logical Operator13/2
  [VDDM_VCURAPSErrLv2_flg] -> Logical Operator13/1
  Logical Operator13/1 -> Switch3/1
